simulink model "Task2"  (R2025a)
settings: Solver=FixedStepAuto  StartTime=0.0  StopTime=10.0  FixedStep=1e-3  MaxStep=1e-3  RelTol=1e-3
settings Model: Creator=LOQ  LastModifiedBy=LOQ

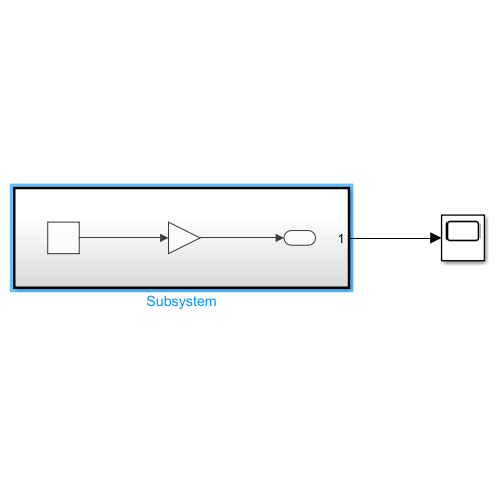
[thumbnail: Simulink's stored preview of the top-level diagram]
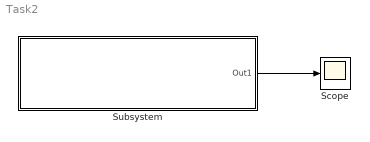
== system Task2 ==
  Scope : Scope
      settings: ActiveDisplayYMinimum=-1  ActiveDisplayYMaximum=1
  Subsystem : Subsystem  TreatAsAtomicUnit=on  SystemSampleTime=0.5
  wires:
  Subsystem/1(Out1) -> Scope/1

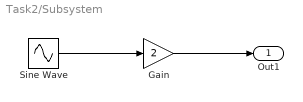
== system Task2/Subsystem ==
  Gain : Gain  Gain=2
  Sine Wave : Sin  SampleTime=0.5
  Out1 : Outport
  wires:
  Sine Wave/1 -> Gain/1
  Gain/1 -> Out1/1
